simulink subsystem "thermal_pipe"  (R2024b)
settings: Solver=VariableStepAuto  StartTime=0.0  StopTime=10.0  RelTol=1e-3
model mask{m_min=0.1, insulation_class=4, D=0.1, L=0, T_duct=15}
  mask prompts: m_min "m_min: non-zero velocity mass flow (for dt=10s, see function doc) [kg/s]"; insulation_class "Thermal insulation class"; D "Pipe diameter [m]"; L "Pipe length [m]"; T_duct "Surrounding temperature [°C]"
settings Model: Creator=nerotb  LastModifiedBy=nerotb

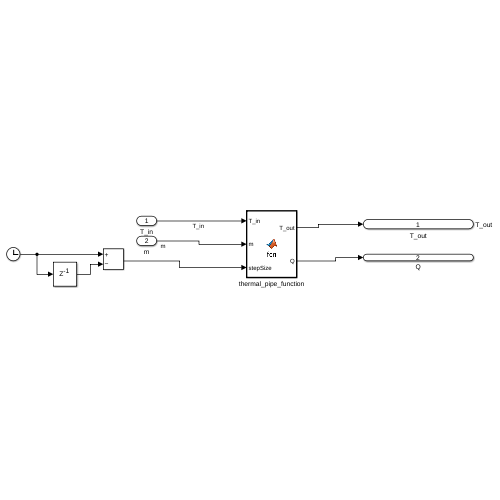
[thumbnail: Simulink's stored preview of the top-level diagram]
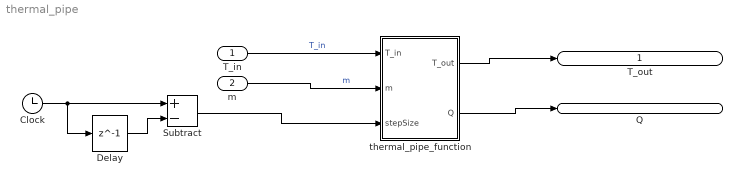
== system thermal_pipe ==
  T_in : Inport
  m : Inport  Port=2
  Clock : Clock
  Delay : Delay  DelayLength=1  InputProcessing=Columns as channels (frame based)
  Subtract : Sum  Inputs=+-
  thermal_pipe_function : MATLAB Function  TreatAsAtomicUnit=on
  T_out : Outport  SignalName=T_out
  Q : Outport  Port=2
  wires:
  T_in/1 -> thermal_pipe_function/1(T_in)  "T_in"
  m/1 -> thermal_pipe_function/2(m)  "m"
  Delay/1 -> Subtract/2
  Clock/1 -> Subtract/1, Delay/1
  Subtract/1 -> thermal_pipe_function/3(stepSize)
  thermal_pipe_function/1(T_out) -> T_out/1
  thermal_pipe_function/2(Q) -> Q/1

== matlab function thermal_pipe/thermal_pipe_function ==
  data: T_out output size=1; T_in input size=1; m input size=1; stepSize input size=1; T_duct parameter size=1; D parameter size=1; L parameter size=1; Q output size=1; insulation_class parameter size=1; m_min parameter size=1
function [T_out, Q]  = fcn(T_in, m, stepSize, T_duct, D, L, insulation_class, m_min)
%% Summary
% This function models a pipe with water entering at temperature T_in and
% exiting at temperature T_out.
% The following effects are taken into account:
%   - delay of propagation of water through the pipe
%   - thermal losses during this propagation time
%
% See the "About m_min" section before use.

%% Model
% Thermal exchange occurs between the water and the surrounding environment 
% at temperature T_duct.
% The pipe is discretized in a 1D mesh along its length.


%% About m_min
% The size of the mesh is determined by `m_min`. 
% `m_min` is the minimum mass flow `m` for water to move in the pipe.
%
% - if m > m_min: the temperatures distribution varies due to both 
% nonzero velocity of the flow and thermal exchange with the duct
% - if m < m_min: the flow is motionless in the pipe, 
% but thermal exchange with the pipe still occurs
%
% A low `m_min` creates a fine mesh, coming with higher algorithmic
% complexity.
%
% m_min is defined for a macro time step of dt_=10 seconds. 
%   If you use a larger time step dt and want to use a m_min value m_min(@dt), 
%   then provide m_min as:
%      m_min = m_min(@dt_) = C * (dt / dt_) * m_min(@dt) 
%                          = C * (dt / 10)  * m_min(@dt)
% For some discreet effects reasons in the meshing definition, 
% it is recommended to apply a safety coefficient C = 0.6.

%% About the macro time step
% For the same reasons as the storage_TC component, 
% macro time step must be constant during the simulation.


%% Parameters
% insulation_class: one of {1, 2, 3, 4, 5, 6}.
%   Defines the k coefficient describing thermal losses per unit meter of
%   pipe [W/(m.K)]. The higher the insulation_class the lower k the better
%   thermal insulation.
%   source: "La conception des réseaux bouclés d'eau chaude sanitaire",ADEME, pages 33 and 111-114
%
% D: diameter of the pipe [m]
% L: length of the pipe [m]
% T_duct: surrounding environment temperature [°C]
% m_min: minimum mass flow for the water not to stagnate within the pipe [kg/s]

%% Variables
% Q: exchanged thermal power, i.e. thermal loss or gain within surrounding air at temperature T_duct [W]
% m: mass flow circulating in the pipe [kg/s]
% T_in: entering temperature of the flow [°C]
% T_out: exiting temperature of the flow [°C]
%   if m > 0: computed as the temporal average over the ode solving duration (=macro time step)
%          of the temperature of the last node (i.e. end of the pipe, where water exits)
%   if m <= 0: temperature of the last node at the end of the ode solving
%       

%% Hypothesis
% - The thermal exchange occurs without any change in temperature at the vicinity of the radiators (T_duct).
% - Cp is constant
% - the thickness of the pipe is 7mm (without thermal insulation)

%% Initialization
% At simulation start, the temperature profile along the pipe is uniform
% with value T_duct.

%% Algorithmic complexity:
% There are:
%   - n variables (temperature distribution along the pipe)
%   - n equations 
%
% The smaller m_min the larger n.


persistent k
persistent T
persistent rho
persistent tau
persistent A
persistent timeIdx    % index of macro time step, starts at 1
persistent oldStepSize
persistent n_dx       % number of meshing nodes
persistent dx         % length of the node [m]



if isempty(k)
    % insulation_class: declared as "Non tunable" for C-code generation compatibility
    % k ~ 0.1 W/(K.m)
    e_pipe = 0.007;
    D_ext = D + 2 * e_pipe;
    if insulation_class == 1
        k = 3.3 * D_ext + 0.22;
    elseif insulation_class == 2
        k = 2.6 * D_ext + 0.20;
    elseif insulation_class == 3
        k = 2 * D_ext + 0.18;
    elseif insulation_class == 4
        k = 1.5 * D_ext + 0.16;
    elseif insulation_class == 5
        k = 1.1 * D_ext + 0.14;
    else % insulation_class == 6
        k = 0.8 * D_ext + 0.12;
    end


    Cp = 4180;
    A = pi * D * D / 4;      % section [m2]
    rho = 1000;
    oldStepSize = -1;
    timeIdx = 1;
    tau = (rho * A * Cp) / k;

    % meshing of pipe:
    % the length of a node (dx) is the distance the water flow covers at the velocity V_min during a duration dt_=10s
    % --> dt_ is independant from the real macro time step because this time step is unknown at first call of the function (see oldStepSize)
    % --> if water velocity is V < V_min, it is set to 0 (equivalent to m=0)

    dt_ = 10;
    V_min = m_min / (rho * A);
    dx_ = V_min * dt_;
    n_dx = floor(L / dx_);  
    n_dx = max(n_dx, 1);    
    dx = L / n_dx;           

    T = ones(1, n_dx) * T_duct;
    
else
    timeIdx = timeIdx + 1;
end


if timeIdx == 1                 
    % initial stepSize value (0) is wrong, 
    % it is replaced by a reasonnable value
    stepSize = 30;
elseif timeIdx == 2
    oldStepSize = stepSize;
else
    assert(abs(oldStepSize - stepSize) < 1e-3) % could be replaced by a call to `isapprox` 
                                               % but this function is not compatible with C-code generation
end


dt = stepSize;    

% m_min is redefined given real macro time step
V_min = dx / dt;
m_min = V_min * rho * A;


if m < 0
    fprintf("Thermal pipe: mass flow m=%1.2e kg/s < 0, it is replaced by zero.\n", m);
    m = 0;
elseif (0 < m) && (m <= m_min)
    fprintf("Thermal pipe: mass flow m=%1.2e kg/s too small for the meshing (m_min value (for dt=%1.1fs): %1.2e kg/s), " + ...
        "it is replaced by zero.\n", m, dt, m_min);
    m = 0;
end


V = m / (rho * A);      % velocity in the pipe [m/s]

t0 = 0;
tf = stepSize;


function out=ODE(t, y, V, T_in)

    % y = [T1, ... , Tn]        n values
    out = zeros(n_dx, 1);

    % node 1
    out(1) =     - (V/dx + 1/tau) * y(1) + 1/tau * T_duct + V * T_in / dx;

    % node i: 2 to n
    for i=2:n_dx
        out(i) = - (V/dx + 1/tau) * y(i) + 1/tau * T_duct + V * y(i-1) / dx;
    end

end


tspan = t0:tf;
options = odeset('RelTol',1e-3, 'AbsTol', 1e-3);
y0 = T;
[~,y] = ode23(@(t, y) ODE(t, y, V, T_in), tspan, y0, options); 

Q = k * L * (mean(y, "all") - T_duct);
T_out = mean(y(:, end));
T = y(end, :);

end
